simulink model "Spreading_effect_frequency_domain"  (Simulink 8.7)
settings: Solver=ode45  StartTime=0.0  StopTime=inf  RelTol=1e-3
undefined symbols (not defined in the file or in its folder): gcbh, rcfiltgaincompat
libraries: commfilt2 x2, commrandsrc2 x1, commseqgen2 x1, commdigbbndam3 x1, commutil2 x1
settings Model: Creator=hongtae  LastModifiedBy=Administrator
settings DataIOCC: SignalLoggingSaveFormat=ModelDataLogs
settings OptimizationCC: ExpressionDepthLimit=2147483647  InitFltsAndDblsToZero=on
settings DebuggingCC: SaveWithParameterizedLinksMsg=none  SignalResolutionControl=TryResolveAllWithWarning  SolverPrmCheckMsg=warning  MultiTaskDSMMsg=warning  MultiTaskCondExecSysMsg=none  FcnCallInpInsideContextMsg=UseLocalSettings  StateNameClashWarn=warning
settings GRTTargetCC: TargetFcnLib=ansi_tfl_tmw.mat  CombineOutputUpdateFcns=off  GRTInterface=on

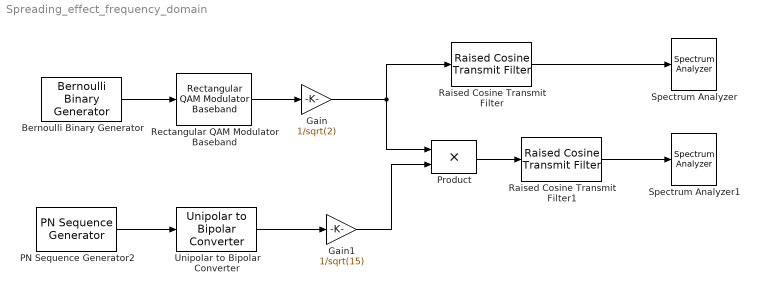
== system Spreading_effect_frequency_domain ==
  Bernoulli Binary Generator : commrandsrc2/Bernoulli Binary Generator  P=0.5  seed=61  Ts=1e-3/2  frameBased=on  sampPerFrame=2  orient=off  outDataType=double
  Gain : Gain  Gain=1/sqrt(2)  SaturateOnIntegerOverflow=on
  Gain1 : Gain  Gain=1/sqrt(15)  SaturateOnIntegerOverflow=on
  PN Sequence Generator2 : commseqgen2/PN Sequence Generator  poly=[1 1 0 0 1]  ini_sta=[0 0 0 1]  outBitMaskSource=Dialog parameter  shift=0  outVarSiz=off  maxOutSizeMode=Dialog parameter  maxOutSize=[10 1]  Ts=1e-3/15  frameBased=on  sampPerFrame=15  reset=off  bitPackedOutputs=off  outDataType=double  numPackedBits=8  bitPackDataSigned=off  bitPackedOutDType=double
  "Product " : Product  SaturateOnIntegerOverflow=on  InputSameDT=on  OutDataTypeStr=Inherit: Same as first input
  Raised Cosine Transmit Filter : commfilt2/Raised Cosine Transmit Filter  filtType=Normal  R=0  filtSpan=2*(4)  N=30  filterGain=rcfiltgaincompat(gcbh)  InputProcessing=Columns as channels (frame based)  RateOptions=Enforce single-rate processing  framing=Mute  checkCoeff=off  variableName=rcTxFilt  checkGain=Normalized  sampMode=Mute  saveAsFlag=0  currentFiltSpan=2*(4)  D=4  launchFVT=off  roundingMode=Floor  overflowMode=off  coeffDataTypeStr=Inherit: Same word length as input  coeffMin=[]  coeffMax=[]  coeffLastDataTypeStr=Inherit: Same word length as input  outputDataTypeStr=Inherit: Same as accumulator  outputMin=[]  outputMax=[]  outputLastDataTypeStr=Inherit: Same as accumulator
  Raised Cosine Transmit Filter1 : commfilt2/Raised Cosine Transmit Filter  filtType=Normal  R=0  filtSpan=2*(4)  N=2  filterGain=rcfiltgaincompat(gcbh)  InputProcessing=Columns as channels (frame based)  RateOptions=Enforce single-rate processing  framing=Mute  checkCoeff=off  variableName=rcTxFilt1  checkGain=Normalized  sampMode=Mute  saveAsFlag=0  currentFiltSpan=2*(4)  D=4  launchFVT=off  roundingMode=Floor  overflowMode=off  coeffDataTypeStr=Inherit: Same word length as input  coeffMin=[]  coeffMax=[]  coeffLastDataTypeStr=Inherit: Same word length as input  outputDataTypeStr=Inherit: Same as accumulator  outputMin=[]  outputMax=[]  outputLastDataTypeStr=Inherit: Same as accumulator
  Rectangular QAM Modulator Baseband : commdigbbndam3/Rectangular QAM Modulator Baseband  M=4  InType=Bit  Enc=Gray  Mapping=[0:15]  PowType=Min. distance between symbols  MinDist=2  AvgPow=1  PeakPow=1  Ph=0  outDtype=double  outWordLen=16  outUDDataType=sfix(16)  outFracLenMode=Best precision  outFracLen=15  outDataTypeStr=double  outLastDataTypeStr=double
  Spectrum Analyzer : SpectrumAnalyzer
  Spectrum Analyzer1 : SpectrumAnalyzer
  Unipolar to Bipolar Converter : commutil2/Unipolar to Bipolar Converter  M=2  polarity=Positive  dataType=Same as input
  wires:
  Gain/1 -> Raised Cosine Transmit Filter/1, "Product "/1
  Gain1/1 -> "Product "/2
  Unipolar to Bipolar Converter/1 -> Gain1/1
  Rectangular QAM Modulator Baseband/1 -> Gain/1
  Bernoulli Binary Generator/1 -> Rectangular QAM Modulator Baseband/1
  PN Sequence Generator2/1 -> Unipolar to Bipolar Converter/1
  Raised Cosine Transmit Filter/1 -> Spectrum Analyzer/1
  "Product "/1 -> Raised Cosine Transmit Filter1/1
  Raised Cosine Transmit Filter1/1 -> Spectrum Analyzer1/1
